simulink model "rotorbroken_gamma"  (R2023a)
settings: Solver=VariableStepAuto  StartTime=0.0  StopTime=2  RelTol=1e-3
libraries: spsACVoltageSourceLib x3, spsAsynchronousMachineSIUnitsLib x1, spsGroundLib x1, spsIdealSwitchLib x1, spsThreePhaseVIMeasurementLib x1, spsdq0toabcLib x1, sps_lib x1, spsSeriesRLCBranchLib x1
settings Model: Creator=user  LastModifiedBy=hp
settings DataIOCC: ReturnWorkspaceOutputs=off

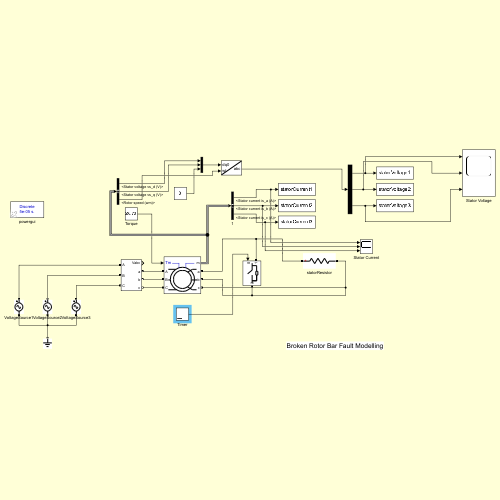
[thumbnail: Simulink's stored preview of the top-level diagram]
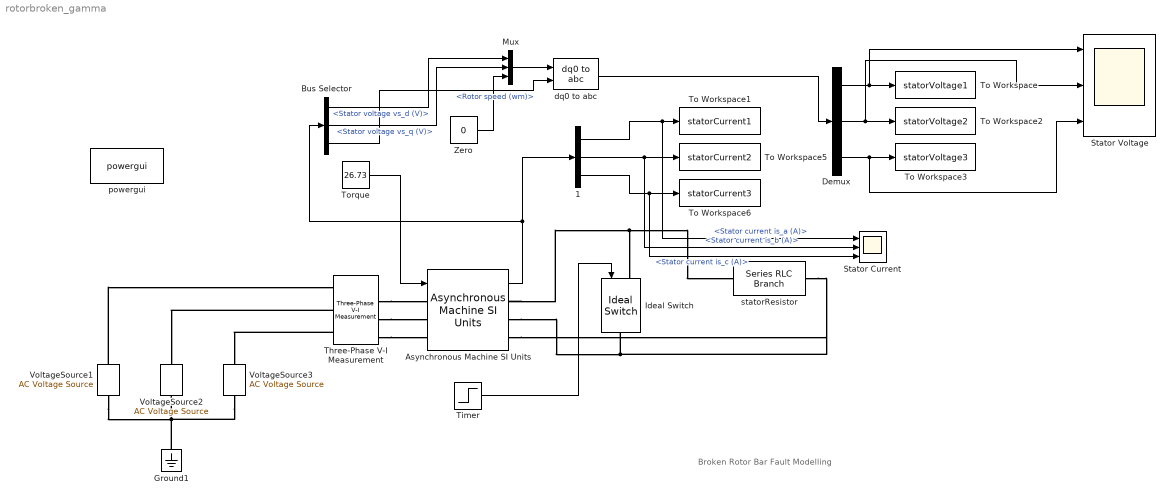
== system rotorbroken_gamma ==
  note: Broken Rotor Bar Fault Modelling
  1 : BusSelector  OutputSignals=Stator measurements.Stator current is_a (A),Stator measurements.Stator current is_b (A),Stator measurements.Stator current is_c (A)
  Asynchronous Machine SI Units : spsAsynchronousMachineSIUnitsLib/Asynchronous Machine SI Units  RotorType=Wound  PresetModel="15:  5.4 HP (4KW)   400 V  50Hz 1430 RPM"  MechanicalLoad=Torque Tm  ShowDetailedParameters=on  ReferenceFrame=Rotor  Units=SI  MeasurementBus=off  NominalParameters=[1.845e+04 400 50]  VoltageRatio=1  Stator=[0.5968 0.0003495]  Rotor=[0.6258 0.005473]  Cage1=[0.4155 0.002066]  Cage2=[0.4168 0.0003495]  Lm=0.0354  Mechanical=[0.05 0.005879 2]  PolePairs=2  InitialConditions=[0 0 0 0 0 0 0 0]  SimulateSaturation=off  Saturation=[14.03593122, 27.81365428, 53.79336849, 72.68890987, 97.98006896, 148.6815601, 215.7428561, 302.9841135, 428.7778367 ; 230, 322, 414, 460, 506, 552, 598, 644, 690]  LoadFlowParameters=1492000  TsPowergui=0  TsBlock=-1  IterativeModel=Trapezoidal non iterative  IterativeDiscreteModel=Trapezoidal non iterative  Pmec=1.492e+006
  Bus Selector : BusSelector  OutputSignals=Stator measurements.Stator voltage vs_d (V),Stator measurements.Stator voltage vs_q (V),Mechanical.Rotor speed (wm)
  Demux : Demux  Outputs=3
  Ground1 : spsGroundLib/Ground  LConnTagsString=a
  Ideal Switch : spsIdealSwitchLib/Ideal Switch  Ron=0.001  Lon=0  IC=1  Rs=1e5  Cs=inf  Measurements=off
  Mux : Mux  Inputs=3
  Stator Current : Scope  NumInputPorts=3
  Stator Voltage : Scope  NumInputPorts=3
  Three-Phase V-I Measurement : spsThreePhaseVIMeasurementLib/Three-Phase V-I Measurement  VoltageMeasurement=phase-to-ground  SetLabelV=off  LabelV=Vabc  Vpu=off  VpuLL=off  CurrentMeasurement=no  SetLabelI=off  LabelI=Iabc  Ipu=off  Pbase=100e6  Vbase=500e3  OutputType=Complex  PhasorSimulation=off  PSBequivalent=0
  Timer : Step  Time=10  SampleTime=0
  To Workspace : ToWorkspace  VariableName=statorVoltage1  SampleTime=-1
  To Workspace1 : ToWorkspace  VariableName=statorCurrent1  SampleTime=-1
  To Workspace2 : ToWorkspace  VariableName=statorVoltage2  SampleTime=-1
  To Workspace3 : ToWorkspace  VariableName=statorVoltage3  SampleTime=-1
  To Workspace5 : ToWorkspace  VariableName=statorCurrent2  SampleTime=-1
  To Workspace6 : ToWorkspace  VariableName=statorCurrent3  SampleTime=-1
  Torque : Constant  Value=26.73
  VoltageSource1 : spsACVoltageSourceLib/AC Voltage Source  Amplitude=224.4444  Phase=0  Frequency=50  SampleTime=0  Measurements=None  BusType=swing  Pref=10e3  Qref=0  Qmin=-inf  Qmax=+inf
  VoltageSource2 : spsACVoltageSourceLib/AC Voltage Source  Amplitude=224.4444  Phase=120  Frequency=50  SampleTime=0  Measurements=None  BusType=swing  Pref=10e3  Qref=0  Qmin=-inf  Qmax=+inf
  VoltageSource3 : spsACVoltageSourceLib/AC Voltage Source  Amplitude=224.4444  Phase=-120  Frequency=50  SampleTime=0  Measurements=None  BusType=swing  Pref=10e3  Qref=0  Qmin=-inf  Qmax=+inf
  Zero : Constant  Value=0  OutDataTypeStr=Inherit: Inherit via back propagation
  dq0 to abc : spsdq0toabcLib/dq0 to abc  Alignment=90 degrees behind phase A axis
  powergui : sps_lib/powergui  Priority=1  SimulationMode=Discrete  SampleTime=50e-6  frequency=60  Iterations=50  frequencyindice=50  Pbase=100e6  ErrMax=1e-4  UnitsV=kV  UnitsW=MW  buscounter=0  FunctionMessages=off  echomessages=off  EnableUseOfTLC=off  CurrentSourceSwitches=off  DisableSnubberDevices=off  DisableRonSwitches=off  DisableVfSwitches=off  DisplayEquations=off  AutomaticDiscreteSolvers=off  SolverType=Tustin/Backward Euler (TBE)  Interpol=off  ExternalGateDelay=off  methode=off  Ts=100  x0status=blocks  SPID=on  SwTol=0  HookPort=off  NonlinearTolerance=1e-4  nMaxIteration=100  ContinueOnMaxIteration=off  RestoreLinks=warning  ResistiveCurrentMeasurement=off  Frange=[0:2:500]  Ylog=off  Xlog=on  ShowGrid=off  save=off  variable=ZData  structure=0  ZoomFFT=off  StartTime=0.0  cycles=1  DisplayStyle=1  fundamental=60  FreqAxis=off  MaxFrequency=1000  frequencyindicesteady=1  RmsSteady=1  display=off
  statorResistor : spsSeriesRLCBranchLib/Series RLC Branch  LConnTagsString=__new0  RConnTagsString=__new0  BranchType=R  Resistance=2.4525  Inductance=1e-3  SetiL0=off  InitialCurrent=0  Capacitance=1e-6  Setx0=off  InitialVoltage=0  Measurements=None
  wires:
  Torque/1 -> Asynchronous Machine SI Units/1
  Asynchronous Machine SI Units/1 -> Bus Selector/1, 1/1
  Timer/1 -> Ideal Switch/1
  Bus Selector/1 -> Mux/1  "<Stator voltage vs_d (V)>"
  Bus Selector/2 -> Mux/2  "<Stator voltage vs_q (V)>"
  Zero/1 -> Mux/3
  Bus Selector/3 -> dq0 to abc/2  "<Rotor speed (wm)>"
  Mux/1 -> dq0 to abc/1
  dq0 to abc/1 -> Demux/1
  Demux/1 -> Stator Voltage/1, To Workspace/1
  Demux/2 -> Stator Voltage/2, To Workspace2/1
  Demux/3 -> Stator Voltage/3, To Workspace3/1
  1/1 -> Stator Current/1, To Workspace1/1  "<Stator current is_a (A)>"
  1/2 -> Stator Current/2, To Workspace5/1  "<Stator current is_b (A)>"
  1/3 -> Stator Current/3, To Workspace6/1  "<Stator current is_c (A)>"
  connections:
  Asynchronous Machine SI Units/RConn2 -- Asynchronous Machine SI Units/RConn3 -- statorResistor/RConn1 -- Ideal Switch/RConn1
  Asynchronous Machine SI Units/RConn1 -- statorResistor/LConn1 -- Ideal Switch/LConn1
  VoltageSource1/RConn1 -- Three-Phase V-I Measurement/LConn1
  Three-Phase V-I Measurement/LConn2 -- VoltageSource2/RConn1
  Three-Phase V-I Measurement/LConn3 -- VoltageSource3/RConn1
  Three-Phase V-I Measurement/RConn1 -- Asynchronous Machine SI Units/LConn1
  Three-Phase V-I Measurement/RConn2 -- Asynchronous Machine SI Units/LConn2
  Three-Phase V-I Measurement/RConn3 -- Asynchronous Machine SI Units/LConn3
  VoltageSource3/LConn1 -- VoltageSource1/LConn1 -- VoltageSource2/LConn1 -- Ground1/LConn1
